simulink model "complex_with_stateflow"  (Simulink 8.0)
settings: Solver=ode45  StartTime=0.0  StopTime=10.0  RelTol=1e-3
undefined symbols (not defined in the file): Ts
libraries: simulink x2
settings Model: Creator=rstarr  LastModifiedBy=rstarr

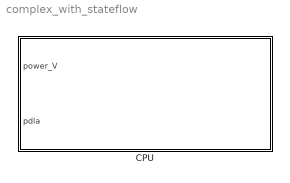
== system complex_with_stateflow ==
  CPU : Subsystem  InitFcn=|  mask(Central Processing Unit){custom_block_type=Cpu, slot_number=0, fixed_slot=off, lower_limit_V=16, upper_limit_V=32, availabilityIndex=1, executionIndex=2, contextIndex=3, parameters_type=Sample based, startingup_time=0, housekeeping_time=0, shuttingdown_time=0, schedule_tasks=off, show_sched_tbl=off}
      | % Get Ts parameter                      
      | Ts =compSys.util.getSimulationStepTime(bdroot(gcbh));
      |                                         
      | updateRtosBlk(gcbh);
      mask prompts: custom_block_type "Custom Block Type"; slot_number "Slot Number"; fixed_slot "Fixed Slot"; lower_limit_V "Power Lower Limit (V):"; upper_limit_V "Power Upper Limit (V):"; availabilityIndex "RTOS Availability Index"; executionIndex "RTOS Execution Index"; contextIndex "RTOS Context Index"; parameters_type "Parameters Type:"; startingup_time "Starting Up Time (number of samples)"; housekeeping_time "House Keeping Time (number of samples)"; shuttingdown_time "Shutting Down Time (number of samples)"; schedule_tasks "Schedule Tasks (click for yes)"; show_sched_tbl "Show Scheduling Table (click for yes)"
      mask help: Processor used in an architectural model.
      mask TypeOptions parameters_type: Sample based | Time based
      mask Display: disp('CPU');

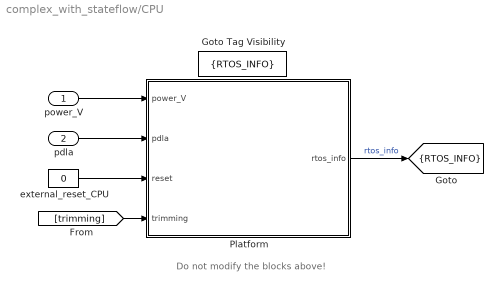
== system complex_with_stateflow/CPU ==
  note: Do not modify the blocks above!
  power_V : Inport
  pdla : Inport  Port=2
  Goto Tag Visibility : GotoTagVisibility  GotoTag=RTOS_INFO
  Platform : Subsystem  Priority=0  mask{custom_block_type=Platform}
      mask prompts: custom_block_type "Custom Block Type"
  external_reset_CPU : Constant  Value=0
  tag scope: RTOS_INFO=scoped
  wires:
  external_reset_CPU/1 -> Platform/3(reset)
  power_V/1 -> Platform/1(power_V)
  pdla/1 -> Platform/2(pdla)
  [trimming] -> Platform/4(trimming)
  Platform/1(rtos_info) -> [RTOS_INFO]  "rtos_info"

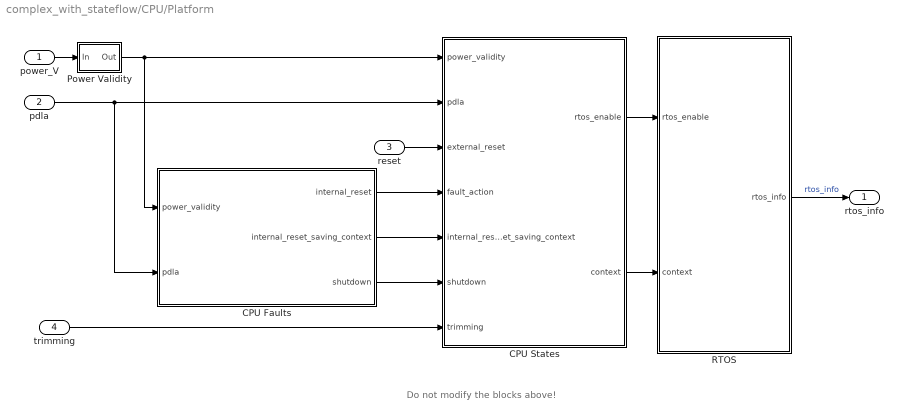
== system complex_with_stateflow/CPU/Platform ==
  note: Do not modify the blocks above!
  power_V : Inport
  pdla : Inport  Port=2
  reset : Inport  Port=3
  trimming : Inport  Port=4
  CPU Faults : Subsystem  mask{custom_block_type=CpuFaults}
      mask prompts: custom_block_type "Custom Block Type"
  CPU States : Subsystem  mask{custom_block_type=CpuStates}
      mask prompts: custom_block_type "Custom Block Type"
  Power Validity : Subsystem
  RTOS : Subsystem  mask{custom_block_type=Rtos, task_quantity=, minor_frame=, minor_frame_info=, minor_frame_quantity=, task_list=, wcetMF=, task_index=}
      mask prompts: custom_block_type "Custom Block Type"; task_quantity "Task Quantity"; minor_frame "Minor Frame (sec)"; minor_frame_info "Minor Frame Information"; minor_frame_quantity "Minor Frame Quantity"; task_list "Task List"; wcetMF "Minor Frame WCET (s)"; task_index "Task Index"
  rtos_info : Outport
  wires:
  trimming/1 -> CPU States/7(trimming)
  CPU States/1(rtos_enable) -> RTOS/1(rtos_enable)
  CPU States/2(context) -> RTOS/2(context)
  reset/1 -> CPU States/3(external_reset)
  RTOS/1(rtos_info) -> rtos_info/1  "rtos_info"
  CPU Faults/1(internal_reset) -> CPU States/4(fault_action)
  CPU Faults/2(internal_reset_saving_context) -> CPU States/5(internal_reset_saving_context)
  CPU Faults/3(shutdown) -> CPU States/6(shutdown)
  power_V/1 -> Power Validity/1(In)
  pdla/1 -> CPU Faults/2(pdla), CPU States/2(pdla)
  Power Validity/1(Out) -> CPU Faults/1(power_validity), CPU States/1(power_validity)

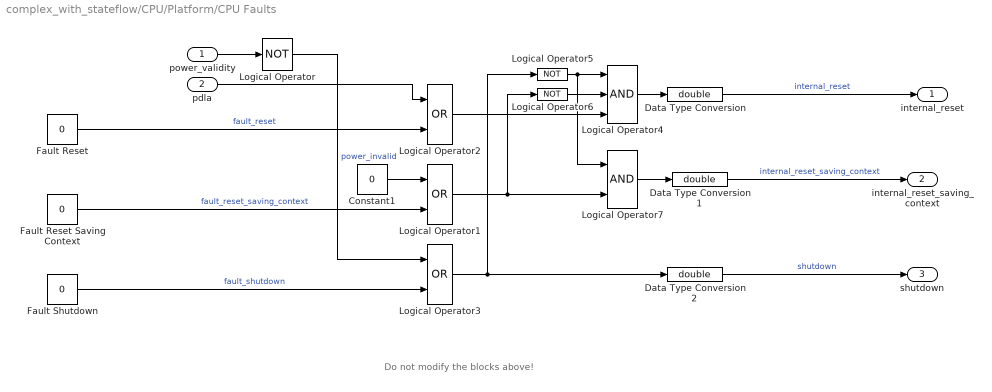
== system complex_with_stateflow/CPU/Platform/CPU Faults ==
  note: Do not modify the blocks above!
  power_validity : Inport
  pdla : Inport  Port=2
  Constant1 : Constant  Value=0
  Data Type Conversion : DataTypeConversion  OutDataTypeStr=double
  Data Type Conversion1 : DataTypeConversion  OutDataTypeStr=double
  Data Type Conversion2 : DataTypeConversion  OutDataTypeStr=double
  Fault Reset : Constant  Value=0
  Fault Reset Saving Context : Constant  Value=0
  Fault Shutdown : Constant  Value=0
  Logical Operator : Logic  Operator=NOT  AllPortsSameDT=off  OutDataTypeStr=boolean
  Logical Operator1 : Logic  Operator=OR  AllPortsSameDT=off  OutDataTypeStr=boolean
  Logical Operator2 : Logic  Operator=OR  AllPortsSameDT=off  OutDataTypeStr=boolean
  Logical Operator3 : Logic  Operator=OR  AllPortsSameDT=off  OutDataTypeStr=boolean
  Logical Operator4 : Logic  Inputs=3  AllPortsSameDT=off  OutDataTypeStr=boolean
  Logical Operator5 : Logic  Operator=NOT  AllPortsSameDT=off  OutDataTypeStr=boolean
  Logical Operator6 : Logic  Operator=NOT  AllPortsSameDT=off  OutDataTypeStr=boolean
  Logical Operator7 : Logic  AllPortsSameDT=off  OutDataTypeStr=boolean
  internal_reset : Outport
  internal_reset_saving_context : Outport  Port=2
  shutdown : Outport  Port=3
  wires:
  Fault Shutdown/1 -> Logical Operator3/2  "fault_shutdown"
  Fault Reset Saving Context/1 -> Logical Operator1/2  "fault_reset_saving_context"
  Fault Reset/1 -> Logical Operator2/2  "fault_reset"
  Logical Operator2/1 -> Logical Operator4/3
  Logical Operator1/1 -> Logical Operator6/1, Logical Operator7/2
  Logical Operator3/1 -> Logical Operator5/1, Data Type Conversion2/1
  Constant1/1 -> Logical Operator1/1
  Logical Operator/1 -> Logical Operator3/1  "power_invalid"
  Logical Operator5/1 -> Logical Operator4/1, Logical Operator7/1
  Logical Operator6/1 -> Logical Operator4/2
  Logical Operator4/1 -> Data Type Conversion/1
  Logical Operator7/1 -> Data Type Conversion1/1
  Data Type Conversion/1 -> internal_reset/1  "internal_reset"
  Data Type Conversion1/1 -> internal_reset_saving_context/1  "internal_reset_saving_context"
  Data Type Conversion2/1 -> shutdown/1  "shutdown"
  power_validity/1 -> Logical Operator/1
  pdla/1 -> Logical Operator2/1

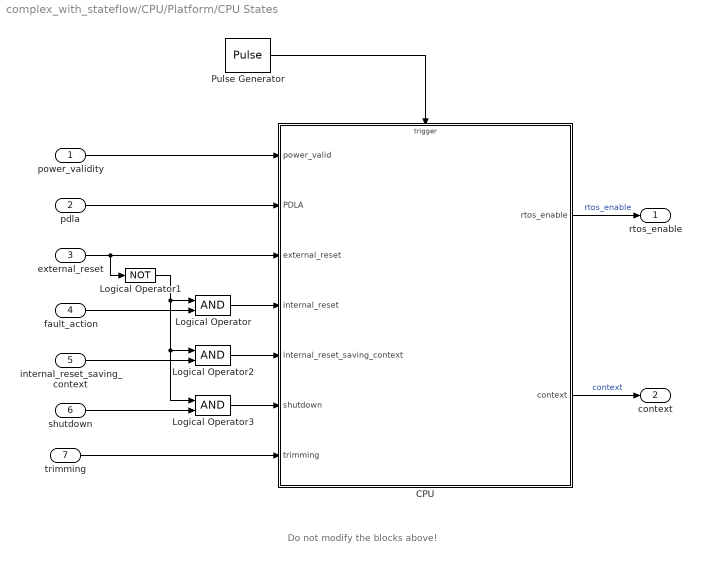
== system complex_with_stateflow/CPU/Platform/CPU States ==
  note: Do not modify the blocks above!
  power_validity : Inport
  pdla : Inport  Port=2
  external_reset : Inport  Port=3
  fault_action : Inport  Port=4
  internal_reset_saving_context : Inport  Port=5
  shutdown : Inport  Port=6
  trimming : Inport  Port=7
  CPU : Stateflow chart  TreatAsAtomicUnit=on
  Logical Operator : Logic  AllPortsSameDT=off  OutDataTypeStr=boolean
  Logical Operator1 : Logic  Operator=NOT  AllPortsSameDT=off  OutDataTypeStr=boolean
  Logical Operator2 : Logic  AllPortsSameDT=off  OutDataTypeStr=boolean
  Logical Operator3 : Logic  AllPortsSameDT=off  OutDataTypeStr=boolean
  Pulse Generator : DiscretePulseGenerator  SampleTime=Ts
  rtos_enable : Outport
  context : Outport  Port=2
  wires:
  trimming/1 -> CPU/7(trimming)
  CPU/1(rtos_enable) -> rtos_enable/1  "rtos_enable"
  CPU/2(context) -> context/1  "context"
  external_reset/1 -> Logical Operator1/1, CPU/3(external_reset)
  Logical Operator1/1 -> Logical Operator/1, Logical Operator2/1, Logical Operator3/1
  fault_action/1 -> Logical Operator/2
  Logical Operator/1 -> CPU/4(internal_reset)
  Logical Operator2/1 -> CPU/5(internal_reset_saving_context)
  Logical Operator3/1 -> CPU/6(shutdown)
  internal_reset_saving_context/1 -> Logical Operator2/2
  shutdown/1 -> Logical Operator3/2
  Pulse Generator/1 -> CPU/Trigger
  power_validity/1 -> CPU/1(power_valid)
  pdla/1 -> CPU/2(PDLA)

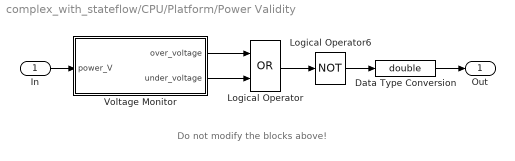
== system complex_with_stateflow/CPU/Platform/Power Validity ==
  note: Do not modify the blocks above!
  In : Inport
  Data Type Conversion : DataTypeConversion  OutDataTypeStr=double
  Logical Operator : Logic  Operator=OR  AllPortsSameDT=off  OutDataTypeStr=boolean
  Logical Operator6 : Logic  Operator=NOT  AllPortsSameDT=off  OutDataTypeStr=boolean
  Voltage Monitor : Subsystem
  Out : Outport
  wires:
  Logical Operator6/1 -> Data Type Conversion/1
  Logical Operator/1 -> Logical Operator6/1
  Voltage Monitor/1(over_voltage) -> Logical Operator/1
  Voltage Monitor/2(under_voltage) -> Logical Operator/2
  Data Type Conversion/1 -> Out/1
  In/1 -> Voltage Monitor/1(power_V)

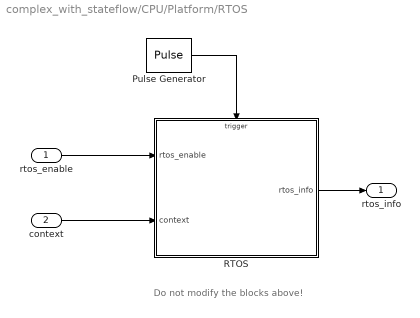
== system complex_with_stateflow/CPU/Platform/RTOS ==
  note: Do not modify the blocks above!
  rtos_enable : Inport
  context : Inport  Port=2
  Pulse Generator : DiscretePulseGenerator  SampleTime=Ts
  RTOS : Stateflow chart  TreatAsAtomicUnit=on
  rtos_info : Outport
  wires:
  Pulse Generator/1 -> RTOS/Trigger
  context/1 -> RTOS/2(context)
  RTOS/1(rtos_info) -> rtos_info/1
  rtos_enable/1 -> RTOS/1(rtos_enable)

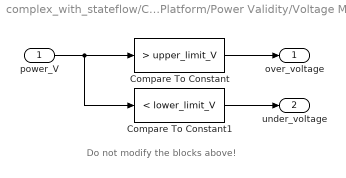
== system complex_with_stateflow/CPU/Platform/Power Validity/Voltage Monitor ==
  note: Do not modify the blocks above!
  power_V : Inport
  Compare To Constant : simulink/Logic and Bit Operations/Compare To Constant  relop=>  const=upper_limit_V  OutDataTypeStr=boolean  ZeroCross=off
  Compare To Constant1 : simulink/Logic and Bit Operations/Compare To Constant  relop=<  const=lower_limit_V  OutDataTypeStr=boolean  ZeroCross=off
  over_voltage : Outport
  under_voltage : Outport  Port=2
  wires:
  Compare To Constant1/1 -> under_voltage/1
  Compare To Constant/1 -> over_voltage/1
  power_V/1 -> Compare To Constant/1, Compare To Constant1/1

== stateflow chart CPU/Platform/CPU States/CPU ==
  settings: executeAtInitialization=1
  state On
    state StartingUp
    state UpAndRunning
      en:
      context = context_action;
      rtos_enable = 1;
    state HouseKeeping
    (default) -> StartingUp
    StartingUp -> UpAndRunning [order 2] : CLK[trimming==1]
    StartingUp -> UpAndRunning [order 1] : after(startingup_time,CLK)
    UpAndRunning -> HouseKeeping : CLK [internal_reset_saving_context == 1]
  state PoweredDown
    en:
    rtos_enable = 0;
  state ShuttingDown
    en:
    rtos_enable = 0;
  (default) -> PoweredDown : {context_action = 1;}
  PoweredDown -> On : CLK [power_valid==1 & PDLA == 0 & internal_reset == 0 &...
      | external_reset == 0 & shutdown == 0 & internal_reset_saving_context  == 0]
  On -> PoweredDown [order 2] : CLK [shutdown == 1]/context_action = 1;
  ShuttingDown -> PoweredDown : after(shuttingdown_time,CLK)
  On -> ShuttingDown [order 1] : CLK [external_reset == 1 | internal_reset == 1]/context_action = 1;
  HouseKeeping -> ShuttingDown : after(housekeeping_time,CLK)/context_action = 2;
  data: rtos_enable output double; power_valid input double; context output double; context_action local double; startingup_time parameter double; shuttingdown_time parameter double; housekeeping_time parameter double; PDLA input double; external_reset input double; internal_reset input double; internal_reset_saving_context input double; shutdown input double; trimming input double size=1
  events: CLK input EITHER_EDGE_EVENT

== stateflow chart CPU/Platform/RTOS/RTOS ==
  settings: executeAtInitialization=1
  state Off
  state On
    en:
    minor_frame_counter = 0;
    defineContext(context);
    ex:
    terminateExecution();
    resetTaskAvailability();
    informTasks();
    state MinorFramePointer
      en:
      minor_frame_counter = minor_frame_counter + 1;
      defineExecution(minor_frame_counter);
      informTasks();
    state NextMinorFrameWaiting
      en:
      resetContext();
      terminateExecution();
      informTasks();
    MinorFramePointer -> NextMinorFrameWaiting : CLK
    (default) -> MinorFramePointer
    NextMinorFrameWaiting -> MinorFramePointer : after((minor_frame/Ts)-1,CLK)
  (default) -> Off
  On -> Off : CLK [rtos_enable == 0]
  Off -> On : CLK [rtos_enable == 1]
  data: context_status function_input double; minor_frame_index function_input double; rtos_enable input double; context input double; rtos_info output double size=[task_quantity_max , 3]; rtos_info_aux local double size=[task_quantity_max, 3]; contextIndex parameter double; executionIndex parameter double; minor_frame_counter local double; Ts parameter double; minor_frame_info parameter double size=[minor_frame_quantity_max, task_quantity_max]; availabilityIndex parameter double; minor_frame_quantity parameter double; task_quantity parameter double; minor_frame parameter double; minor_frame_quantity_max constant double =50; task_quantity_max constant double =50
  events: CLK input EITHER_EDGE_EVENT
  function defineContext(context_status):
    | %*************************************************************************
    | % Function defineContext updates the context information
    | % with the "context_status" variable content.
    | %*************************************************************************
    | % The "context_status" variable may assume one of the following values 
    | % 0 (reset task context) or 1 (do not reset task context).
    | %*************************************************************************
    | 
    | function defineContext(context_status)
    | 
    |     % for each existing task
    |     % update the context column (whose index corresponds to "restoreIndex" 
    |     % variable) of the temporary variable rtos_info_aux with 
    |     % the "context_status" variable content 
    |     rtos_info_aux(:,contextIndex) = context;    
    | 
    | end
  function resetTaskAvailability:
    | %*************************************************************************
    | % Function resetTaskAvailability updates the availability
    | % os each task to 0 (unavailable)
    | %*************************************************************************
    | 
    | function resetTaskAvailability()
    |      
    |     rtos_info_aux(:,availabilityIndex) = 0;  
    |   
    | end
  function defineExecution(minor_frame_index):
    | %*************************************************************************
    | % Function defineExecution seraches the Scheduling Table for the nonzero 
    | % values, that correspond to the task ids that shall be executed
    | %*************************************************************************
    | 
    | function defineExecution(minor_frame_index)
    | 
    |     % Find modulus after dividing minor_frame_index (equal to minor_frame_counter value, initially zero)
    |     % by minor_frame_quantity
    |     minor_frame_index = mod(minor_frame_index, minor_frame_quantity);
    | 
    |     % If minor_frame_index is a multiple of minor_frame_quantity
    |     if minor_frame_index == 0
    |         % Index cannot be zero, set it with the minor_frame_quantity value
    |         minor_frame_index = minor_frame_quantity;
    |     end;
    | 
    |     % For each task
    |     for minor_frame_sequence = 1:task_quantity
    |         % Get task id from Scheduling Table position: row = minor_frame_index, 
    |         % column = minor_frame_sequence
    |          task_id = minor_frame_info(minor_frame_index,minor_frame_sequence);
    |          % If Scheduling Table position is filled with a task id (value different from zero)
    |          if task_id ~= 0
    |              % Update auxiliary Scheduling Table execution column with 1 (disable task)
    |              rtos_info_aux(task_id,executionIndex) = 1;
    |              rtos_info_aux(task_id,availabilityIndex) = 1;
    |          end;
    |     end;
    | 
    | end
  function terminateExecution:
    | %*************************************************************************
    | % Function terminateExecution stop the execution of all tasks
    | %*************************************************************************
    | 
    | function terminateExecution()
    |  
    |     % Disable task execution
    |     rtos_info_aux(:,executionIndex) = 0;   
    | end
  function resetContext:
    | %*************************************************************************
    | % Function resetContext set the context to 0 for each task 
    | % that was executed. The value 0 indicated that the context 
    | % has to be maintained. 
    | % Notes: context = 1 (to reset the context) and context = 2 (to restore 
    | % the context previously saved).
    | %*************************************************************************
    | 
    | function resetContext
    |  
    |     % For all tasks
    |     for i = 1:task_quantity
    |         if(rtos_info_aux(i,executionIndex) == 1)
    |             % Freeze context
    |             rtos_info_aux(i,contextIndex) = 0;
    |         end
    |     end;
    | end
  function informTasks:
    | %*************************************************************************
    | % Function informTasks sends the information (availability, context and
    | %execution), which were prepared in RTOS, to the tasks.
    | %*************************************************************************
    | 
    | function informTasks
    |     rtos_info = rtos_info_aux;   
    | end
